simulink model "linear"  (R2022b)
settings: Solver=VariableStepAuto  StartTime=0.0  StopTime=10.0  RelTol=1e-3
values from neighbouring files (symbols this model uses):
  A = [0 1 0 0; 0 0 m*g/M 0; 0 0 0 1; 0 0 (M+m)*g/(M*l) 0]    [invertpen_script.m]
  B = [0;1/M;0;1/l/M]    [invertpen_script.m]
  C = [1,0,0,0;0,0,1,0]    [invertpen_script.m]
  D = [0;0]    [invertpen_script.m]
  K = -1*SF_controller_1    [invertpen_script.m]
undefined symbols (not defined in the file or in its folder): I, L, x_init
settings Model: Creator=kevin  LastModifiedBy=kevin

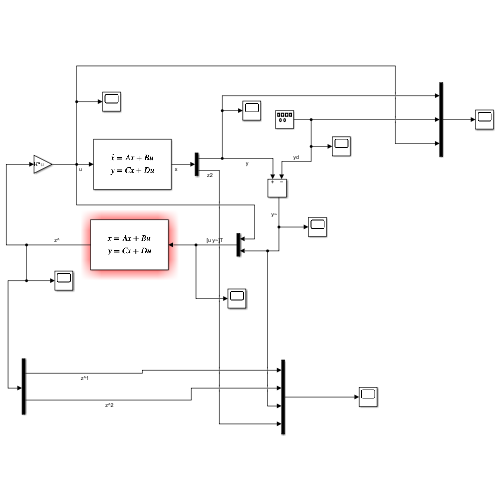
[thumbnail: Simulink's stored preview of the top-level diagram]
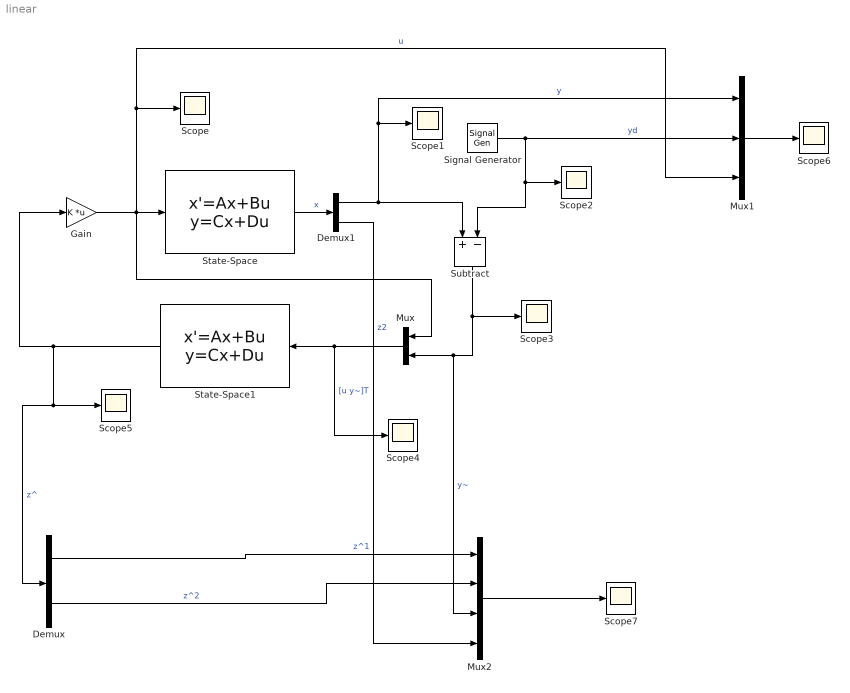
== system linear ==
  Demux : Demux  Outputs=2
  Demux1 : Demux  Outputs=2
  Gain : Gain  Gain=K  Multiplication=Matrix(K*u)
  Mux : Mux  Inputs=2
  Mux1 : Mux  Inputs=3
  Mux2 : Mux
  Scope{,1..7} (8 alike) : Scope
  Signal Generator : SignalGenerator  WaveForm=square  Amplitude=0.015  Frequency=0.5
  State-Space : StateSpace  A=A  B=B  C=C  D=D  InitialCondition=x_init
  State-Space1 : StateSpace  A=A-L*C  B=[B L]  C=I  D=[0 0; 0 0]  InitialCondition=[0; 0]
  Subtract : Sum  Inputs=+-
  wires:
  Demux/2 -> Mux2/2  "z^2"
  Signal Generator/1 -> Mux1/2, Scope2/1, Subtract/2  "yd"
  State-Space1/1 -> Demux/1, Scope5/1, Gain/1  "z^"
  Demux1/1 -> Subtract/1, Mux1/1, Scope1/1  "y"
  State-Space/1 -> Demux1/1  "x"
  Demux1/2 -> Mux2/4  "z2"
  Mux2/1 -> Scope7/1
  Mux1/1 -> Scope6/1
  Subtract/1 -> Scope3/1, Mux2/3, Mux/2  "y~"
  Demux/1 -> Mux2/1  "z^1"
  Gain/1 -> Scope/1, Mux1/3, Mux/1, State-Space/1  "u"
  Mux/1 -> Scope4/1, State-Space1/1  "[u y~]T"
